simulink model "ARDroneHover"  (R2018b)
settings: Solver=ode1  StartTime=0.0  StopTime=inf  FixedStep=sampleTime  RelTol=1e-3  EnableMultiTasking=on
values from neighbouring files (symbols this model uses):
  sampleTime = 0.01    [setupHover.m]    (also in setupTT.m; setupWPTracking.m)
undefined symbols (not defined in the file or in its folder): DiscIntNeverNeededParam, Standard_Devices, UDP_Protocol
libraries: hdlsllib x6, dspnetwork x4, sldrtlib x3, simulink x1
(part 2 of 2)

== matlab function ARDroneHover/Outer-loop Controller/MATLAB Function ==
  data: w_r output; dot_psi_r output; theta_r output; states input; pd input; dot_pd input; ddot_pd input; psi_d input; xi input; phi_r output; dot_xi output
function [w_r, dot_psi_r, theta_r, phi_r, dot_xi] = tt_controller(states, pd, dot_pd, ddot_pd,psi_d,xi)
%#codegen

% ------------------------------------------------------------------------
% inputs:
% states - structure with state variables
% pd - desired position
% dot_pd - desired velocity
% ddot_pt - desired acceleration
% psi_d - desired yaw angle
% xi - integral state (four variables)
%
% outputs:
% w_r - vertical velocity reference
% dot_psi_r - yaw rate reference
% theta_r - pitch angle reference
% phi_r - roll angle reference
% dot_xi - integral state derivative
% ------------------------------------------------------------------------

lambda = states(1:3,1); % Euler angles
psi = lambda(3);
R=euler2R(lambda);
Rz = [cos(psi) -sin(psi) 0; sin(psi) cos(psi) 0; 0 0 1];
psi_e = normalize_angle(psi-psi_d);

p = states(7:9,1); % position vector
p(3) = -p(3); % height is symmetric of z

vb = states(4:6,1);
dot_p = R*vb; % body velocity rotated to inertial frame 
dot_p(3) = -dot_p(3);

%!!!!!!!!!!!!!!!!!!!!!!!!!!!!!!!!!!!!!!!!!!!!!!!!!!!!!!!!!!!!!!!!!!!!!!
% replace with the necessary code to implement the trajectory tracking
% controller
w_r= 0;
dot_psi_r = 0;
theta_r = 0;
phi_r = 0;
dot_xi = [0;0;0;0];
%!!!!!!!!!!!!!!!!!!!!!!!!!!!!!!!!!!!!!!!!!!!!!!!!!!!!!!!!!!!!!!!!!!!!!!

k1=1;
k2=2;
k3=0;
x_e = [p-pd; dot_p-dot_pd];
K = [k1*eye(3) k2*eye(3)];

g=9.81;
e3=[0;0;1];
% integrator in inertial frame
u_star = Rz'*(K*x_e + g*e3 - ddot_pd + xi(1:3,1));
% integrator in body frame
%u_star = Rz'*(K*x_e + g*e3 - ddot_pd + R*xi(1:3,1));

w_r = -(-p(3)-(-pd(3)));
dot_psi_r = -1.5*psi_e-0*xi(4);
theta_r = atan2(u_star(1),u_star(3));
phi_r = atan2(-u_star(2),sqrt(u_star(1)^2 + u_star(3)^2));
% integrator in inertial frame
dot_xi = [k3*K*x_e;psi_e];
% integrator in body frame
%dot_xi = [k3*k1*R'*(p-pd);psi_e];
%dot_xi = [k3*(p-pd);psi_e];


function R = euler2R(l)
%#codegen
% returns the rotation matrix for a given vector of euler angles

phi = l(1); theta = l(2); psi = l(3);
R = [cos(theta)*cos(psi)...
      sin(phi)*sin(theta)*cos(psi)-cos(phi)*sin(psi)...
      cos(phi)*sin(theta)*cos(psi)+sin(phi)*sin(psi);
   cos(theta)*sin(psi)...
   sin(phi)*sin(theta)*sin(psi)+cos(phi)*cos(psi)... 
   cos(phi)*sin(theta)*sin(psi)-sin(phi)*cos(psi);
   -sin(theta)...
   sin(phi)*cos(theta)...
   cos(phi)*cos(theta)];

function angleOut = normalize_angle(angleIn)
%#codegen

angleOut = mod(angleIn, 2*pi) ;
if angleOut > pi
    angleOut = -2*pi + angleOut ; 
end

== matlab function ARDroneHover/Data to States/Compute the Derivative/MATLAB Function ==
  data: u input; y output
function y = ZOH_nan(u)

persistent u_

if isempty(u_)
    u_ = 0;
end

if isnan(u)
    u = u_;
else
    u_ = u;
end

y = u;

== matlab function ARDroneHover/Data to States/Compute the Derivative/MATLAB Function1 ==
  data: u input; y output
function y = ZOH_nan(u)

persistent u_

if isempty(u_)
    u_ = 0;
end

if isnan(u)
    u = u_;
else
    u_ = u;
end

y = u;

== matlab function ARDroneHover/Data to States/Compute the Derivative/MATLAB Function2 ==
  data: u input; y output
function y = ZOH_nan(u)

persistent u_

if isempty(u_)
    u_ = 0;
end

if isnan(u)
    u = u_;
else
    u_ = u;
end

y = u;

== matlab function ARDroneHover/Data from Qualisys/Subsystem/MATLAB Function1 ==
  data: x4 output uint8; x3 output uint8; x2 output uint8; data input; x1 output uint8; object input
function [x4,x3,x2,x1] = fcn(data,object)

slot=(object-1)*8;

x1=data(41+slot);
x2=data(41+slot+1);
x3=data(41+slot+2);
x4=data(41+slot+3);

== matlab function ARDroneHover/Data from Qualisys/Subsystem/MATLAB Function2 ==
  data: x input uint32 size=1; X output single size=1; y input; Y output; z input; roll input; pitch input; yaw input; Z output; Roll output; Pitch output; Yaw output
function [X,Y,Z,Roll,Pitch,Yaw] = fcn(x,y,z,roll,pitch,yaw)


X = typecast(uint32(x),'single');
Y = typecast(uint32(y),'single');
Z = typecast(uint32(z),'single');
Roll = typecast(uint32(roll),'single');
Pitch = typecast(uint32(pitch),'single');
Yaw = typecast(uint32(yaw),'single');

== matlab function ARDroneHover/Data from Qualisys/Subsystem/MATLAB Function3 ==
  data: y4 output uint8; y3 output uint8; y2 output uint8; data input; y1 output uint8; object input
function [y4,y3,y2,y1] = fcn(data,object)

slot=(object-1)*8;

y1=data(45+slot);
y2=data(45+slot+1);
y3=data(45+slot+2);
y4=data(45+slot+3);

== matlab function ARDroneHover/Data from Qualisys/Subsystem/MATLAB Function4 ==
  data: z4 output uint8; z3 output uint8; z2 output uint8; data input; z1 output uint8; object input
function [z4,z3,z2,z1] = fcn(data,object)

slot=(object-1)*8;

z1=data(49+slot);
z2=data(49+slot+1);
z3=data(49+slot+2);
z4=data(49+slot+3);

== matlab function ARDroneHover/Data from Qualisys/Subsystem/MATLAB Function5 ==
  data: roll4 output uint8; roll3 output uint8; roll2 output uint8; data input; roll1 output uint8; object input
function [roll4,roll3,roll2,roll1] = fcn(data,object)

slot=(object-1)*8;

roll1=data(53+slot);
roll2=data(53+slot+1);
roll3=data(53+slot+2);
roll4=data(53+slot+3);

== matlab function ARDroneHover/Data from Qualisys/Subsystem/MATLAB Function6 ==
  data: pitch4 output uint8; pitch3 output uint8; pitch2 output uint8; data input; pitch1 output uint8; object input
function [pitch4,pitch3,pitch2,pitch1] = fcn(data,object)

slot=(object-1)*8;

pitch1=data(57+slot);
pitch2=data(57+slot+1);
pitch3=data(57+slot+2);
pitch4=data(57+slot+3);

== matlab function ARDroneHover/Data from Qualisys/Subsystem/MATLAB Function7 ==
  data: yaw4 output uint8; yaw3 output uint8; yaw2 output uint8; data input; yaw1 output uint8; object input
function [yaw4,yaw3,yaw2,yaw1] = fcn(data,object)

slot=(object-1)*8;

yaw1=data(61+slot);
yaw2=data(61+slot+1);
yaw3=data(61+slot+2);
yaw4=data(61+slot+3);

== matlab function ARDroneHover/Data to States/MATLAB Function ==
  data: v input; v_b output; phi input; theta input; psi input
function v_b = fcn(v,phi,theta,psi)

R = [cos(theta)*cos(psi)...
      sin(phi)*sin(theta)*cos(psi)-cos(phi)*sin(psi)...
      cos(phi)*sin(theta)*cos(psi)+sin(phi)*sin(psi);
   cos(theta)*sin(psi)...
   sin(phi)*sin(theta)*sin(psi)+cos(phi)*cos(psi)... 
   cos(phi)*sin(theta)*sin(psi)-sin(phi)*cos(psi);
   -sin(theta)...
   sin(phi)*cos(theta)...
   cos(phi)*cos(theta)];

v_b = R'*v;

== matlab function ARDroneHover/MATLAB Function1 ==
  data: on_off input; states input; t input; pd output; dot_pd output; ddot_pd output; psi_d output
function [pd, dot_pd, ddot_pd, psi_d] = desired_trajectory(on_off,states,t)
%#codegen

% ------------------------------------------------------------------------
% inputs:
% on_off - 1 if tracking is on, 0 if it is off
% states - structure with state variables
% t - current simulation time
% 
% outputs:
% pd - desired position
% dot_pd - desired velocity
% ddot_pd - desired acceleration
% psi_d - desired yaw angle
% ------------------------------------------------------------------------

persistent t0
persistent p0
persistent previous_status

on = 1;
off = 0;

if isempty(previous_status)
    previous_status = on;
    p0 = [states(7:8);-1];
end

if on_off == off
    if previous_status == on 
    % first time off or switching back off
        p0 = [states(7:8);-1]; % x0 and y0 match the current position
    end
    pd = p0;
    dot_pd = [0;0;0];
    ddot_pd = [0;0;0];
    psi_d = 0;
else
    if isempty(t0) || (previous_status == off) 
    % first time on or switching back on
        t0 = t;
        p0 = [states(7:8);-1];
    end
    dt = t-t0;

%!!!!!!!!!!!!!!!!!!!!!!!!!!!!!!!!!!!!!!!!!!!!!!!!!!!!!!!!!!!!!!!!!!!!!!!!
% replace with the necessary code to define adequate desired trajectories
% use dt, p0, and any additional parameters
%     pd = p0;
%     dot_pd = [0;0;0];
%     ddot_pd = [0;0;0];
%     psi_d = 0;
% 
    om = 0.5;
    pd = p0 + [cos(om*dt)-1;sin(om*dt);0];%[0.5*dt;0;0];
    dot_pd = om*[-sin(om*dt);cos(om*dt);0];%[0.5;0;0];
    ddot_pd = om^2*[-cos(om*dt);-sin(om*dt);0];%[0;0;0];
    psi_d = om*dt;

%     pd = p0 + [0.5*dt;0;0];
%     dot_pd = [0.5;0;0];
%     ddot_pd = [0;0;0];
%     psi_d = 0;
%     
%     if pd(1) > 1
%         pd(1) = 1;
%         dot_pd(1) = 0;
%     end
    
%     Delta = 0.5;
%     V = 1;
%     psi_d = atan2(-(states(8)-1),Delta);
%     dot_psi_d = -states(5)/Delta/(1+((states(8)-1)/Delta)^2);
%     dot_pd = V*[cos(psi_d);sin(psi_d);0];
%     ddot_pd = V*dot_psi_d*[-sin(psi_d);cos(psi_d);0];
%     pd = [states(7:8);-1];
%     psi_d = 0;

%!!!!!!!!!!!!!!!!!!!!!!!!!!!!!!!!!!!!!!!!!!!!!!!!!!!!!!!!!!!!!!!!!!!!!!!!

end

previous_status = on_off;
